simulink model "SecondOrderOverdampedSystemSimulink"  (R2023b)
settings: Solver=VariableStepAuto  StartTime=0.0  StopTime=10.0  RelTol=1e-3
undefined symbols (not defined in the file): G_den1, G_num1
settings Model: Creator=Emanuel  LastModifiedBy=Emanuel

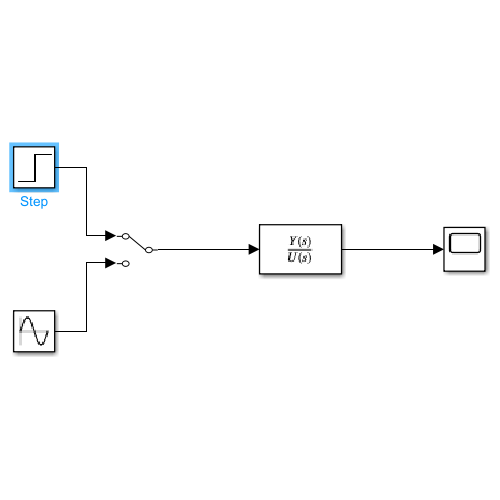
[thumbnail: Simulink's stored preview of the top-level diagram]
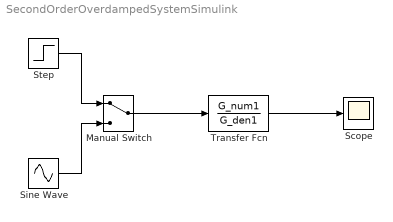
== system SecondOrderOverdampedSystemSimulink ==
  Manual Switch : ManualSwitch
  Scope : Scope
  Sine Wave : Sin  SampleTime=0
  Step : Step  Time=0  SampleTime=0
  Transfer Fcn : TransferFcn  Numerator=G_num1  Denominator=G_den1
  wires:
  Step/1 -> Manual Switch/1
  Sine Wave/1 -> Manual Switch/2
  Manual Switch/1 -> Transfer Fcn/1
  Transfer Fcn/1 -> Scope/1
